simulink model "Linear_Control_Lab_Lab6_ServoMotor_Position_Control_2"  (R2018b)
settings: Solver=VariableStepAuto  StartTime=0.0  StopTime=30.0  RelTol=1e-3
settings Model: Creator=HP  LastModifiedBy=HP

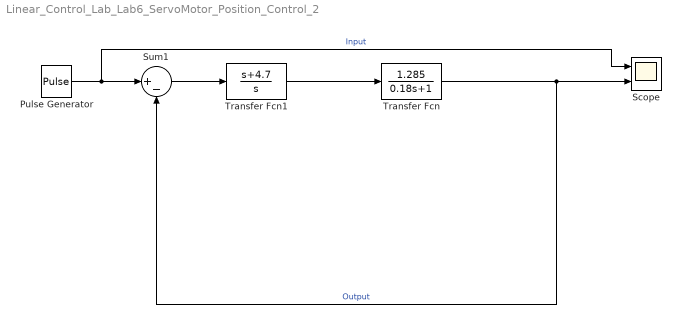
== system Linear_Control_Lab_Lab6_ServoMotor_Position_Control_2 ==
  Pulse Generator : DiscretePulseGenerator  PulseType=Time based  Amplitude=3  Period=10  PulseWidth=50
  Scope : Scope  NumInputPorts=2
  Sum1 : Sum  Inputs=|+-
  Transfer Fcn : TransferFcn  Numerator=[1.285]  Denominator=[0.18 1]
  Transfer Fcn1 : TransferFcn  Numerator=[1 4.7]  Denominator=[1 0]
  wires:
  Pulse Generator/1 -> Scope/1, Sum1/1  "Input"
  Transfer Fcn/1 -> Scope/2, Sum1/2  "Output"
  Sum1/1 -> Transfer Fcn1/1
  Transfer Fcn1/1 -> Transfer Fcn/1
